simulink model "perturbaciones"  (R2020b)
settings: Solver=VariableStepAuto  StartTime=0.0  StopTime=40  RelTol=1e-3
settings Model: Creator=carma  LastModifiedBy=carma

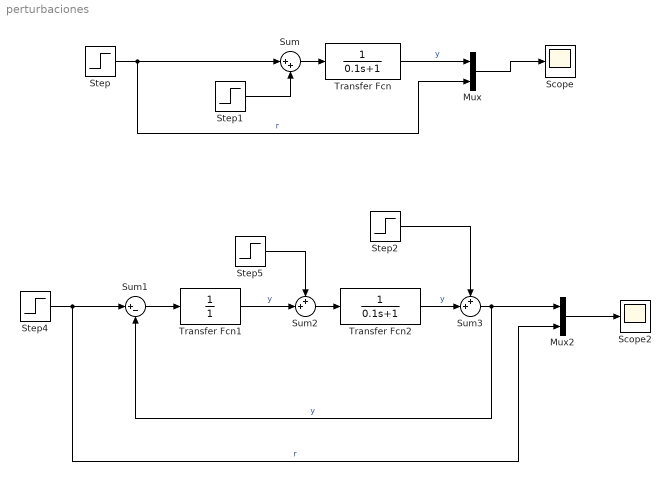
== system perturbaciones ==
  Mux : Mux  Inputs=2
  Mux2 : Mux  Inputs=2
  Scope : Scope
  Scope2 : Scope
  Step : Step  Time=0  SampleTime=0
  Step1 : Step  Time=6  After=0.3  SampleTime=0
  Step2 : Step  Time=16  After=0.1  SampleTime=0
  Step4 : Step  Time=0  SampleTime=0
  Step5 : Step  Time=6  After=0.3  SampleTime=0
  Sum : Sum  Inputs=|++
  Sum1 : Sum  Inputs=|+-
  Sum2 : Sum  Inputs=++|
  Sum3 : Sum  Inputs=++|
  Transfer Fcn : TransferFcn  Denominator=[0.1 1]
  Transfer Fcn1 : TransferFcn  Denominator=[1]
  Transfer Fcn2 : TransferFcn  Denominator=[0.1 1]
  wires:
  Sum/1 -> Transfer Fcn/1
  Step/1 -> Mux/2, Sum/1  "r"
  Step1/1 -> Sum/2
  Mux/1 -> Scope/1
  Transfer Fcn/1 -> Mux/1  "y"
  Mux2/1 -> Scope2/1
  Sum2/1 -> Transfer Fcn2/1
  Step4/1 -> Sum1/1, Mux2/2  "r"
  Step5/1 -> Sum2/1
  Sum1/1 -> Transfer Fcn1/1
  Step2/1 -> Sum3/1
  Transfer Fcn2/1 -> Sum3/2  "y"
  Sum3/1 -> Sum1/2, Mux2/1  "y"
  Transfer Fcn1/1 -> Sum2/2  "y"
